simulink model "vision_RPi2_soln"  (R2018a)
settings: Solver=FixedStepAuto  StartTime=0.0  StopTime=inf  RelTol=1e-3  EnableMultiTasking=on
libraries: embdlinuxlib x2, raspberrypilib x1, visiontextngfix x1
settings Model: SimulationMode=external  Creator=cdsouza  LastModifiedBy=scastro
settings SolverCC: PositivePriorityOrder=on
settings OptimizationCC: PassReuseOutputArgsAs=Individual arguments  MaxStackSize=64
settings DebuggingCC: ParameterTunabilityLossMsg=error
settings HardwareCC: ProdBitPerPointer=32  ProdBitPerSizeT=32  ProdBitPerPtrDiffT=32  ProdLargestAtomicInteger=Long  ProdLargestAtomicFloat=Double  ProdWordSize=32  ProdHWDeviceType=ARM Compatible->ARM Cortex
settings SFSimCC: MATLABDynamicMemAlloc=off
settings RTWCC: SystemTargetFile=ert.tlc  HardwareBoard=Raspberry Pi  TLCOptions="-aInlineSetEventsForThisBaseRateFcn=TLC_FALSE -aSuppressMultiTaskScheduler=TLC_FALSE  -aRateBasedStepFcn=0"  TemplateMakefile=ert_default_tmf  GenerateReport=on  Toolchain=GNU GCC Raspberry Pi  IncludeHyperlinkInReport=on  LaunchReport=on  GenerateTraceInfo=on  GenerateTraceReport=on  GenerateTraceReportSl=on  GenerateTraceReportSf=on  GenerateTraceReportEml=on
settings CodeAppCC: ForceParamTrailComments=on  IgnoreCustomStorageClasses=off  OperatorAnnotations=on  SimulinkDataObjDesc=on  SFDataObjDesc=on  InsertBlockDesc=on
settings ERTTargetCC: SupportVariableSizeSignals=on

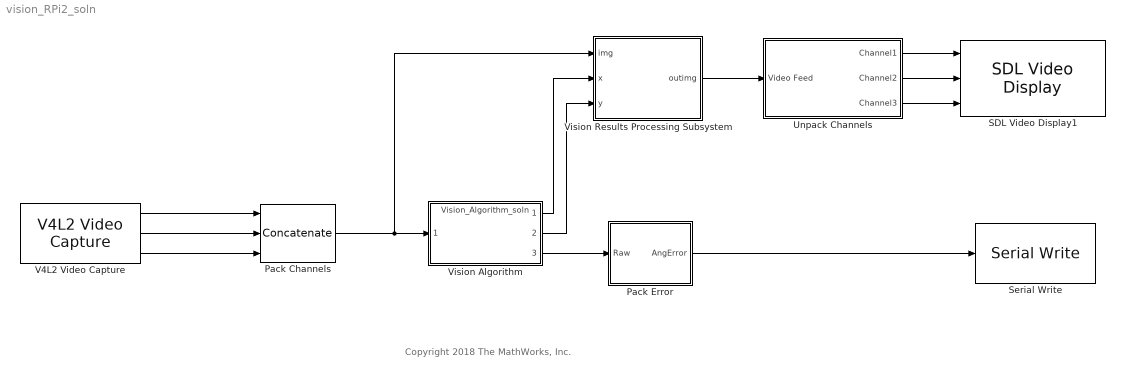
== system vision_RPi2_soln ==
  note: Copyright 2018 The MathWorks, Inc.
  Pack Channels : Concatenate  NumInputs=3  Mode=Multidimensional array  ConcatenateDimension=3
  Pack Error : Subsystem
  SDL Video Display1 : embdlinuxlib/SDL Video Display  pixelFormat=RGB  pixelOrder=Planar  rowMajor=on  blockPlatform=Raspberry Pi
      settings: SourceProductName=Simulink Support Package for Raspberry Pi Hardware  SourceProductBaseCode=RASPPI
  Serial Write : raspberrypilib/Serial Write  board=Pi 3 Model B  SCIModule_=/dev/ttyACM0  Baudrate_=9600  Parity=None  StopBits_=1  HardwareFlowControl=None  ByteOrder=LittleEndian  OutputStatus=off  blockPlatform=RaspberryPi
      settings: SourceProductName=Simulink Support Package for Raspberry Pi Hardware  SourceProductBaseCode=RASPPI
  Unpack Channels : Subsystem
  V4L2 Video Capture : embdlinuxlib/V4L2 Video Capture  m_devName='/dev/video0'  roi=[0, 0, 640, 480]  imSizeSelection=320x240  imSize=[640, 480]  pixelFormat=RGB  pixelOrder=Planar  sampleTime=0.05  simOutput=Colorbars  blockPlatform=Raspberry Pi
      settings: SourceProductName=Simulink Support Package for Raspberry Pi Hardware  SourceProductBaseCode=RASPPI
  Vision Algorithm : ModelReference  ModelNameDialog=Vision_Algorithm_soln.slx  SimulationMode=Normal  ModelReferenceVersion=1.36
  Vision Results Processing Subsystem : Subsystem
  wires:
  Pack Error/1(AngError) -> Serial Write/1
  Vision Algorithm/1 -> Vision Results Processing Subsystem/2(x)
  Vision Algorithm/2 -> Vision Results Processing Subsystem/3(y)
  Vision Algorithm/3 -> Pack Error/1(Raw)
  Unpack Channels/1(Channel1) -> SDL Video Display1/1
  Unpack Channels/2(Channel2) -> SDL Video Display1/2
  Unpack Channels/3(Channel3) -> SDL Video Display1/3
  Vision Results Processing Subsystem/1(outimg) -> Unpack Channels/1(Video Feed)
  Pack Channels/1 -> Vision Algorithm/1, Vision Results Processing Subsystem/1(img)
  V4L2 Video Capture/2 -> Pack Channels/2
  V4L2 Video Capture/3 -> Pack Channels/3
  V4L2 Video Capture/1 -> Pack Channels/1

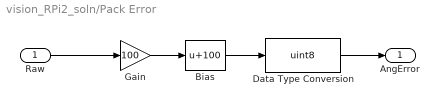
== system vision_RPi2_soln/Pack Error ==
  Raw : Inport
  Bias : Bias  Bias=100
  Data Type Conversion : DataTypeConversion  OutDataTypeStr=uint8
  Gain : Gain  Gain=100
  AngError : Outport
  wires:
  Data Type Conversion/1 -> AngError/1
  Gain/1 -> Bias/1
  Raw/1 -> Gain/1
  Bias/1 -> Data Type Conversion/1

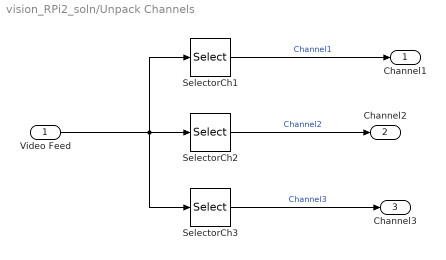
== system vision_RPi2_soln/Unpack Channels ==
  Video Feed : Inport
  SelectorCh1 : Selector  NumberOfDimensions=3  InputPortWidth=3  IndexOptions=Select all,Select all,Index vector (dialog)  Indices=1,1,1  OutputSizes=1,1,1
  SelectorCh2 : Selector  NumberOfDimensions=3  InputPortWidth=3  IndexOptions=Select all,Select all,Index vector (dialog)  Indices=1,2,2  OutputSizes=1,1,1
  SelectorCh3 : Selector  NumberOfDimensions=3  InputPortWidth=3  IndexOptions=Select all,Select all,Index vector (dialog)  Indices=1,1,3  OutputSizes=1,1,1
  Channel1 : Outport
  Channel2 : Outport  Port=2
  Channel3 : Outport  Port=3
  wires:
  SelectorCh3/1 -> Channel3/1  "Channel3"
  SelectorCh1/1 -> Channel1/1  "Channel1"
  SelectorCh2/1 -> Channel2/1  "Channel2"
  Video Feed/1 -> SelectorCh3/1, SelectorCh2/1, SelectorCh1/1

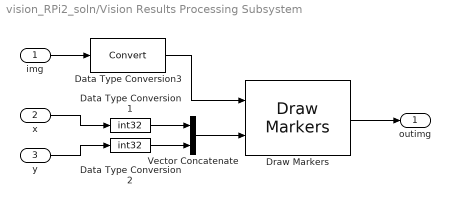
== system vision_RPi2_soln/Vision Results Processing Subsystem ==
  img : Inport
  x : Inport  Port=2
  y : Inport  Port=3
  Data Type Conversion1 : DataTypeConversion  OutDataTypeStr=int32
  Data Type Conversion2 : DataTypeConversion  OutDataTypeStr=int32
  Data Type Conversion3 : DataTypeConversion
  Draw Markers : visiontextngfix/Draw Markers  shape=Circle  size=3  fill=off  fillClrSource=Specify via dialog  display=Black  intensity=200  color=[200 255 100]  opacity=0.6  viewport=Entire image  antialiasing=off  inType=Obsolete  imagePorts=One multidimensional signal  prodOutputMode=Binary point scaling  prodOutputWordLength=32  prodOutputFracLength=14  memoryMode=Specify word length  memoryWordLength=16  memoryFracLength=15  roundingMode=Floor  overflowMode=off
      settings: SourceProductName=Computer Vision System Toolbox  SourceProductBaseCode=VP
  Vector Concatenate : Concatenate
  outimg : Outport
  wires:
  Data Type Conversion3/1 -> Draw Markers/1
  Vector Concatenate/1 -> Draw Markers/2
  Data Type Conversion2/1 -> Vector Concatenate/2
  Draw Markers/1 -> outimg/1
  Data Type Conversion1/1 -> Vector Concatenate/1
  y/1 -> Data Type Conversion2/1
  img/1 -> Data Type Conversion3/1
  x/1 -> Data Type Conversion1/1
